simulink model "aracerMV"  (R2024b)
settings: Solver=FixedStepAuto  StartTime=0.0  StopTime=100  FixedStep=0.01  RelTol=1e-3
libraries: simulink x2
settings Model: Creator=mrdan  LastModifiedBy=mrudi
settings OptimizationCC: DefaultParameterBehavior=Inlined  EnhancedBackFolding=on  PassReuseOutputArgsAs=Individual arguments  ZeroExternalMemoryAtStartup=off  ZeroInternalMemoryAtStartup=off  MaxStackSize=64  OptimizeBlockOrder=speed  DifferentSizesBufferReuse=on  OptimizationCustomize=off  EfficientTunableParamExpr=on
settings DebuggingCC: ParameterTunabilityLossMsg=error
settings HardwareCC: ProdBitPerPointer=32  ProdBitPerSizeT=32  ProdBitPerPtrDiffT=32  ProdLargestAtomicFloat=None  ProdIntDivRoundTo=Undefined  ProdEndianess=Unspecified  ProdWordSize=32  ProdHWDeviceType=Generic->Unspecified (assume 32-bit Generic)  UseEmbeddedCoderFeatures=off
settings SFSimCC: MATLABDynamicMemAlloc=off
settings RTWCC: Description=Embedded Coder  SystemTargetFile=ert.tlc  HardwareBoard=Robot Operating System (ROS)  TLCOptions="-aInlineSetEventsForThisBaseRateFcn=TLC_FALSE -aSuppressMultiTaskScheduler=TLC_FALSE  -aRateBasedStepFcn=0"  GenCodeOnly=on  TemplateMakefile=ert_default_tmf  Toolchain=Catkin  TargetLang=C++
settings CodeAppCC: ForceParamTrailComments=on  IgnoreCustomStorageClasses=off  OperatorAnnotations=on  SimulinkDataObjDesc=on  SFDataObjDesc=on  InsertBlockDesc=on
settings ERTTargetCC: SupportNonInlinedSFcns=on

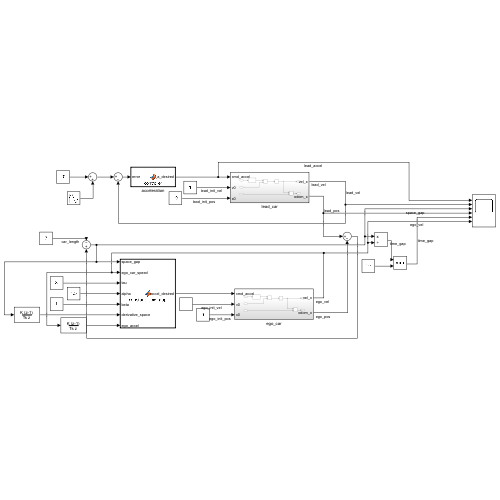
[thumbnail: Simulink's stored preview of the top-level diagram]
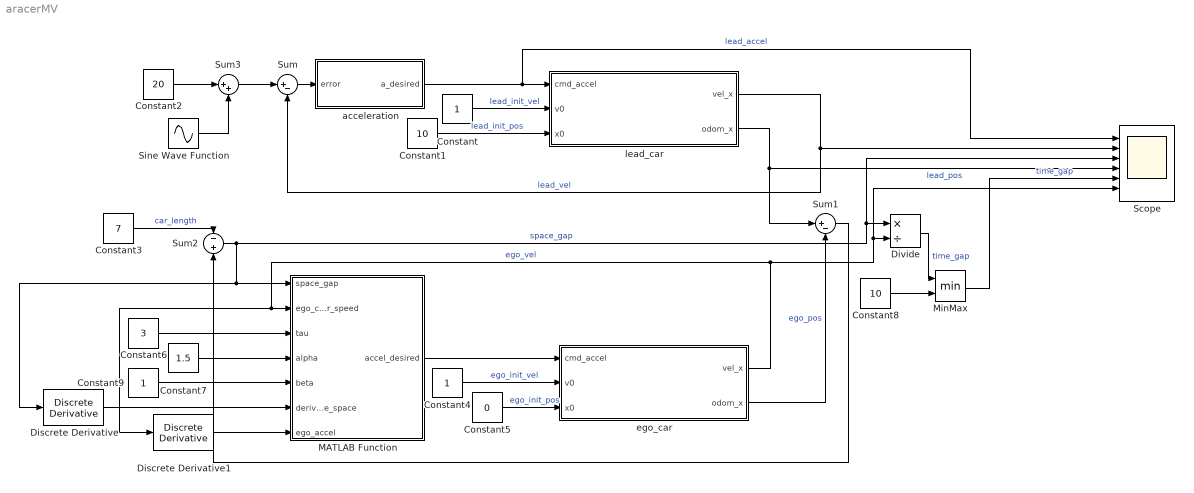
== system aracerMV ==
  Constant : Constant
  Constant1 : Constant  Value=10
  Constant2 : Constant  Value=20
  Constant3 : Constant  Value=7
  Constant4 : Constant
  Constant5 : Constant  Value=0
  Constant6 : Constant  Value=3
  Constant7 : Constant  Value=1.5
  Constant8 : Constant  Value=10
  Constant9 : Constant
  Discrete Derivative : simulink/Discrete/Discrete Derivative  gainval=1.0  ICPrevScaledInput=0.0  OutMin=[]  OutMax=[]  OutDataType=fixdt(1, 16)  OutScaling=2^-10  DoSatur=off
  Discrete Derivative1 : simulink/Discrete/Discrete Derivative  gainval=1.0  ICPrevScaledInput=0.0  OutMin=[]  OutMax=[]  OutDataType=fixdt(1, 16)  OutScaling=2^-10  DoSatur=off
  Divide : Product  Inputs=*/
  MATLAB Function : MATLAB Function  TreatAsAtomicUnit=on
  MinMax : MinMax  Inputs=2
  Scope : Scope  NumInputPorts=6
  Sine Wave Function : Sin  Amplitude=5  SampleTime=0
  Sum : Sum  Inputs=|+-
  Sum1 : Sum  Inputs=|+-
  Sum2 : Sum  Inputs=-+
  Sum3 : Sum  Inputs=|++
  acceleration : MATLAB Function  TreatAsAtomicUnit=on
  ego_car : Subsystem
  lead_car : Subsystem
  wires:
  acceleration/1(a_desired) -> Scope/1, lead_car/1(cmd_accel)  "lead_accel"
  Sum/1 -> acceleration/1(error)
  lead_car/2(odom_x) -> Sum1/1, Scope/4  "lead_pos"
  Constant1/1 -> lead_car/3(x0)  "lead_init_pos"
  Constant/1 -> lead_car/2(v0)  "lead_init_vel"
  lead_car/1(vel_x) -> Sum/2, Scope/2  "lead_vel"
  Constant3/1 -> Sum2/1  "car_length"
  Sum1/1 -> Sum2/2
  Sum2/1 -> Discrete Derivative/1, MATLAB Function/1(space_gap), Divide/1, Scope/3  "space_gap"
  MATLAB Function/1(accel_desired) -> ego_car/1(cmd_accel)
  Constant4/1 -> ego_car/2(v0)  "ego_init_vel"
  Constant5/1 -> ego_car/3(x0)  "ego_init_pos"
  ego_car/2(odom_x) -> Sum1/2  "ego_pos"
  ego_car/1(vel_x) -> Discrete Derivative1/1, MATLAB Function/2(ego_car_speed), Scope/6, Divide/2  "ego_vel"
  Constant6/1 -> MATLAB Function/3(tau)
  Constant7/1 -> MATLAB Function/4(alpha)
  Constant2/1 -> Sum3/1
  Sine Wave Function/1 -> Sum3/2
  Sum3/1 -> Sum/1
  MinMax/1 -> Scope/5  "time_gap"
  Divide/1 -> MinMax/1  "time_gap"
  Constant8/1 -> MinMax/2
  Constant9/1 -> MATLAB Function/5(beta)
  Discrete Derivative/1 -> MATLAB Function/6(derivative_space)
  Discrete Derivative1/1 -> MATLAB Function/7(ego_accel)

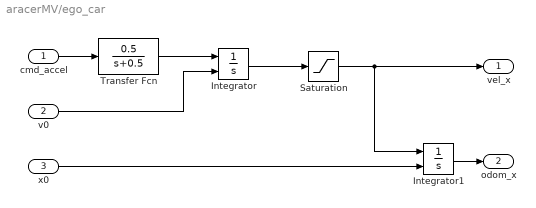
== system aracerMV/ego_car ==
  cmd_accel : Inport
  v0 : Inport  Port=2
  x0 : Inport  Port=3
  Integrator : Integrator  InitialConditionSource=external
  Integrator1 : Integrator  InitialConditionSource=external
  Saturation : Saturate  UpperLimit=80  LowerLimit=0
  Transfer Fcn : TransferFcn  Numerator=[0.5]  Denominator=[1 0.5]
  vel_x : Outport
  odom_x : Outport  Port=2
  wires:
  v0/1 -> Integrator/2
  cmd_accel/1 -> Transfer Fcn/1
  Transfer Fcn/1 -> Integrator/1
  Integrator1/1 -> odom_x/1
  Integrator/1 -> Saturation/1
  x0/1 -> Integrator1/2
  Saturation/1 -> vel_x/1, Integrator1/1

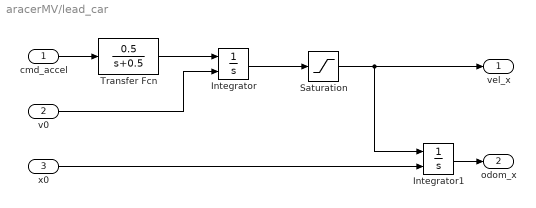
== system aracerMV/lead_car ==
  cmd_accel : Inport
  v0 : Inport  Port=2
  x0 : Inport  Port=3
  Integrator : Integrator  InitialConditionSource=external
  Integrator1 : Integrator  InitialConditionSource=external
  Saturation : Saturate  UpperLimit=80  LowerLimit=0
  Transfer Fcn : TransferFcn  Numerator=[0.5]  Denominator=[1 0.5]
  vel_x : Outport
  odom_x : Outport  Port=2
  wires:
  v0/1 -> Integrator/2
  cmd_accel/1 -> Transfer Fcn/1
  Transfer Fcn/1 -> Integrator/1
  Integrator1/1 -> odom_x/1
  Integrator/1 -> Saturation/1
  x0/1 -> Integrator1/2
  Saturation/1 -> vel_x/1, Integrator1/1

== matlab function aracerMV/MATLAB Function ==
  data: space_gap input; accel_desired output; ego_car_speed input; tau input; alpha input; beta input; derivative_space input; ego_accel input
function accel_desired = constant_time_gap(space_gap, ego_car_speed, tau, alpha, beta, derivative_space, ego_accel)

accel_desired = alpha * (space_gap - tau * ego_car_speed) + beta * (derivative_space - tau * ego_accel);

== matlab function aracerMV/acceleration ==
  data: error input; a_desired output
function a_desired = controller(error)
a_desired = max(-1.5, min(3, error));
end
